simulink model "es2_1_1"  (Simulink 3.00)
settings: Solver=ode45  StartTime=0.0  StopTime=30.0  RelTol=1e-5
values from neighbouring files (symbols this model uses):
  Kc = 1    [es_V.m]
  Kr = 1    [es_V.m]
libraries: cstblocks x1, simulink3 x1

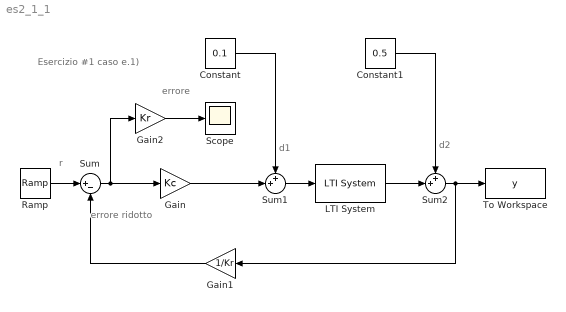
== system es2_1_1 ==
  note: errore
      | ridotto
  note: errore
  note: Esercizio #1
      | caso e.1)
  note: r
  note: d1
  note: d2
  Constant : Constant  Value=0.1
  Constant1 : Constant  Value=0.5
  Gain : Gain  Gain=Kc  SaturateOnIntegerOverflow=on
  Gain1 : Gain  Orientation=left  Gain=1/Kr  SaturateOnIntegerOverflow=on
  Gain2 : Gain  Gain=Kr  SaturateOnIntegerOverflow=on
  LTI System : cstblocks/LTI System  sys=F  IC=[0]
  Ramp : simulink3/Sources/Ramp  slope=1  start=0  X0=0
  Scope : Scope
      settings: TimeRange=auto  YMin=-5  YMax=5  SaveToWorkspace=off  SaveName=ScopeData
  Sum : Sum  Inputs=|+-  SaturateOnIntegerOverflow=on
  Sum1 : Sum  Inputs=++|  SaturateOnIntegerOverflow=on
  Sum2 : Sum  Inputs=++|  SaturateOnIntegerOverflow=on
  To Workspace : ToWorkspace  VariableName=y  SampleTime=-1  SaveFormat=Matrix
  wires:
  Ramp/1 -> Sum/1
  Gain/1 -> Sum1/2
  Gain1/1 -> Sum/2
  Sum/1 -> Gain/1, Gain2/1
  Gain2/1 -> Scope/1
  Constant/1 -> Sum1/1
  Sum1/1 -> LTI System/1
  LTI System/1 -> Sum2/2
  Constant1/1 -> Sum2/1
  Sum2/1 -> To Workspace/1, Gain1/1
